simulink library "INT_InjCrv_MI1Cor"  (R2016b)
settings: Solver=VariableStepAuto  StartTime=0.0  StopTime=10.0  RelTol=1e-3
settings Model: Creator=Administrator  LastModifiedBy=Administrator

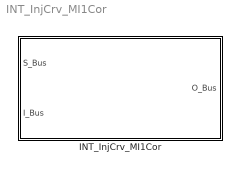
== system INT_InjCrv_MI1Cor ==
  INT_InjCrv_MI1Cor : Subsystem

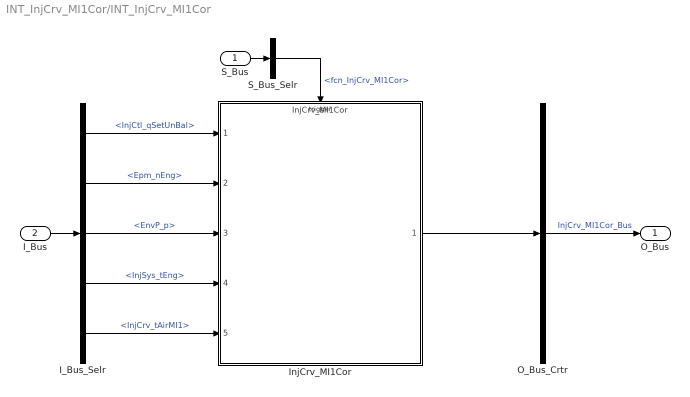
== system INT_InjCrv_MI1Cor/INT_InjCrv_MI1Cor ==
  S_Bus : Inport
  I_Bus : Inport  Port=2
  I_Bus_Selr : BusSelector  OutputSignals=InjCtl_qSetUnBal,Epm_nEng,EnvP_p,InjSys_tEng,InjCrv_tAirMI1
  InjCrv_MI1Cor : ModelReference  ModelNameDialog=InjCrv_MI1Cor  SimulationMode=Normal  ModelReferenceVersion=1.17  TriggerPortName=function  TriggerPortTriggerType=function-call  TriggerPortStatesWhenEnabling=held
  O_Bus_Crtr : BusCreator  Inputs=1
  S_Bus_Selr : BusSelector  OutputSignals=fcn_InjCrv_MI1Cor
  O_Bus : Outport
  wires:
  S_Bus_Selr/1 -> InjCrv_MI1Cor/Trigger  "<fcn_InjCrv_MI1Cor>"
  S_Bus/1 -> S_Bus_Selr/1
  I_Bus/1 -> I_Bus_Selr/1
  I_Bus_Selr/1 -> InjCrv_MI1Cor/1  "<InjCtl_qSetUnBal>"
  I_Bus_Selr/2 -> InjCrv_MI1Cor/2  "<Epm_nEng>"
  I_Bus_Selr/3 -> InjCrv_MI1Cor/3  "<EnvP_p>"
  I_Bus_Selr/4 -> InjCrv_MI1Cor/4  "<InjSys_tEng>"
  I_Bus_Selr/5 -> InjCrv_MI1Cor/5  "<InjCrv_tAirMI1>"
  O_Bus_Crtr/1 -> O_Bus/1  "InjCrv_MI1Cor_Bus"
  InjCrv_MI1Cor/1 -> O_Bus_Crtr/1
